simulink model "svpwmmod"  (R2020a)
settings: Solver=ode1  StartTime=0.0  StopTime=0.05  FixedStep=10e-6  MaxStep=0.00001  RelTol=1e-3
InitFcn:
  | Ualf=250;
  | Ubet=250;
  | f=50;
  | fc=5000;
  | Udc=500;
  | T_dead=20e-4
libraries: powerlib x23, dsparch4 x8, simulink x4, powerlib_meascontrol x2
settings Model: Creator=Administrator  LastModifiedBy=DELL
settings SolverCC: AutoInsertRateTranBlk=on
settings DataIOCC: LimitDataPoints=on  SaveFormat=Array  SignalLoggingSaveFormat=ModelDataLogs  ReturnWorkspaceOutputs=off
settings OptimizationCC: ExpressionDepthLimit=2147483647  InitFltsAndDblsToZero=on  LifeSpan=inf
settings DebuggingCC: SaveWithParameterizedLinksMsg=none  UnderspecifiedInitializationDetection=Classic  MergeDetectMultiDrivingBlocksExec=none  SignalResolutionControl=TryResolveAllWithWarning  SolverPrmCheckMsg=warning  MultiTaskDSMMsg=warning  MultiTaskCondExecSysMsg=none  MultiTaskRateTransMsg=warning  FcnCallInpInsideContextMsg=warning  StateNameClashWarn=warning  SFUnexpectedBacktrackingDiag=warning  SFNoUnconditionalDefaultTransitionDiag=warning  ArithmeticOperatorsInVariantConditions=warning
settings HardwareCC: ProdBitPerPointer=32  ProdBitPerSizeT=32  ProdBitPerPtrDiffT=32  ProdLargestAtomicFloat=None  ProdIntDivRoundTo=Undefined  ProdEndianess=Unspecified  ProdWordSize=32  ProdHWDeviceType=32-bit Generic
settings ModelReferenceCC: PropagateSignalLabelsOutOfModel=off
settings SFSimCC: SimUseLocalCustomCode=off  CustomCodeUndefinedFunction=UseInterfaceOnly
settings RTWCC: RTWUseLocalCustomCode=off
settings CodeAppCC: StateflowObjectComments=on
settings GRTTargetCC: TargetFcnLib=ansi_tfl_tmw.mat  TargetLangStandard=C89/C90 (ANSI)  CombineOutputUpdateFcns=off  GRTInterface=on
settings ConfigComp: CovMetricSettings=dw  CovHtmlReporting=on  CovSaveCumulativeToWorkspaceVar=on  CovSaveSingleToWorkspaceVar=on  CovExternalEMLEnable=off

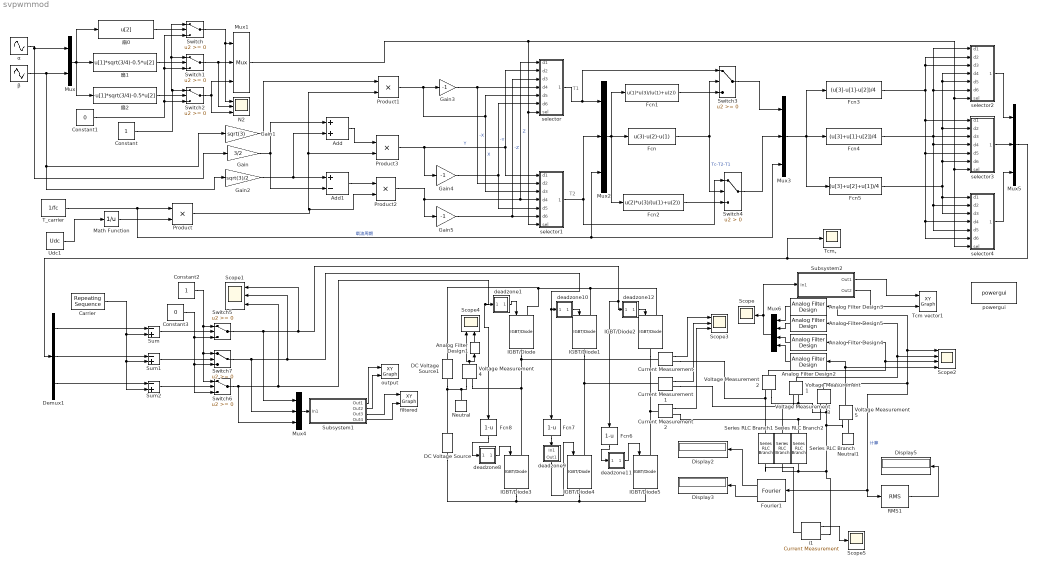
== system svpwmmod ==
  note: T2
  note: T1
  Add : Sum
  Add1 : Sum  Inputs=+-
  Analog Filter Design{1..5} (5 alike) : dsparch4/Analog Filter Design  method=Bessel  filttype=Lowpass  N=4  Wlo=1200  Whi=80  Rp=2  Rs=40
  "Carrier " : simulink/Sources/Repeating Sequence  rep_seq_t=[0 1/(2*fc) 1/(fc)]  rep_seq_y=[0 1/10000 0]
  Constant : Constant
  Constant1 : Constant  Value=0
  Constant2 : Constant
  Constant3 : Constant  Value=0
  Current Measurement : powerlib/Measurements/Current Measurement  PhasorSimulation=off  OutputType=Complex  PSBequivalent=0
  Current Measurement1 : powerlib/Measurements/Current Measurement  PhasorSimulation=off  OutputType=Complex  PSBequivalent=0
  Current Measurement2 : powerlib/Measurements/Current Measurement  PhasorSimulation=off  OutputType=Complex  PSBequivalent=0
  DC Voltage Source : powerlib/Electrical Sources/DC Voltage Source  Amplitude=0.5*(Udc)  Measurements=None
  DC Voltage Source1 : powerlib/Electrical Sources/DC Voltage Source  Amplitude=0.5*(Udc)  Measurements=None
  Demux1 : Demux  Outputs=3
  Display2 : Display
  Display3 : Display
  Display5 : Display
  Fcn : Fcn  Expr=u(3)-u(2)-u(1)
  Fcn1 : Fcn  Expr=u(1)*u(3)/(u(1)+u(2))
  Fcn2 : Fcn  Expr=u(2)*u(3)/(u(1)+u(2))
  Fcn3 : Fcn  Expr=(u[3]-u[1]-u[2])/4
  Fcn4 : Fcn  Expr=(u[3]+u[1]-u[2])/4
  Fcn5 : Fcn  Expr=(u[3]+u[2]+u[1])/4
  Fcn6 : Fcn  Expr=1-u
  Fcn7 : Fcn  Expr=1-u
  Fcn8 : Fcn  Expr=1-u
  Fourier1 : powerlib_meascontrol/Measurements/Fourier  Freq=50  n=1  InInit=[0, 0]  Ts=0
  Gain : Gain  Gain=3/2
  Gain1 : Gain  Gain=sqrt(3)
  Gain2 : Gain  Gain=sqrt(3)/2
  Gain3 : Gain  Gain=-1
  Gain4 : Gain  Gain=-1
  Gain5 : Gain  Gain=-1
  IGBT/Diode{,1..5} (6 alike) : powerlib/Power Electronics/IGBT//Diode  Ron=1e-3  Rs=1e5  Cs=inf  Measurements=off
  Math Function : Math  Operator=reciprocal  SignedPower=on  SaturateOnIntegerOverflow=on
  Mux : Mux  Inputs=2
  Mux{1..5} (5 alike) : Mux  Inputs=3
  Mux6 : Mux
  N2 : Scope  NumInputPorts=3
  Neutral : powerlib/Elements/Neutral  LConnTagsString=a  NodeNumber=10
      settings: SourceProductBaseCode=PS
  Neutral1 : powerlib/Elements/Neutral  LConnTagsString=a  NodeNumber=10
      settings: SourceProductBaseCode=PS
  Product{,1..3} (4 alike) : Product  RndMeth=Zero
  RMS1 : powerlib_meascontrol/Measurements/RMS  TrueRMS=on  Freq=60  RMSInit=120  Ts=0
  Scope : Scope
  Scope1 : Scope  NumInputPorts=3
  Scope2 : Scope  NumInputPorts=4
  Scope3 : Scope  NumInputPorts=3
  Scope4 : Scope  NumInputPorts=2
  Scope5 : Scope
  Series RLC Branch : powerlib/Elements/Series RLC Branch  LConnTagsString=__new0  RConnTagsString=__new0  BranchType=RL  Resistance=10  Inductance=5e-3  SetiL0=off  InitialCurrent=0  Capacitance=1e-6  Setx0=off  InitialVoltage=0  Measurements=None
  Series RLC Branch1 : powerlib/Elements/Series RLC Branch  LConnTagsString=__new0  RConnTagsString=__new0  BranchType=RL  Resistance=10  Inductance=5e-3  SetiL0=off  InitialCurrent=0  Capacitance=1e-6  Setx0=off  InitialVoltage=0  Measurements=None
  Series RLC Branch2 : powerlib/Elements/Series RLC Branch  LConnTagsString=__new0  RConnTagsString=__new0  BranchType=RL  Resistance=10  Inductance=5e-3  SetiL0=off  InitialCurrent=0  Capacitance=1e-6  Setx0=off  InitialVoltage=0  Measurements=None
  Subsystem1 : Subsystem
  Subsystem2 : Subsystem
  Sum : Sum  Inputs=-+  SaturateOnIntegerOverflow=on
  Sum1 : Sum  Inputs=-+  SaturateOnIntegerOverflow=on
  Sum2 : Sum  Inputs=-+  SaturateOnIntegerOverflow=on
  Switch{,1..3} (4 alike) : Switch
  Switch4 : Switch  Criteria=u2 > Threshold
  Switch5 : Switch  SaturateOnIntegerOverflow=on
  Switch6 : Switch  SaturateOnIntegerOverflow=on
  Switch7 : Switch  SaturateOnIntegerOverflow=on
  T_carrier : Constant  Value=1/fc
  Tcm vector1 : simulink/Sinks/XY Graph  xmin=-400  xmax=400  ymin=-400  ymax=400  st=-1
  Tcm。 : Scope
  Udc1 : Constant  Value=Udc
  Voltage Measurement{1..5} (5 alike) : powerlib/Measurements/Voltage Measurement  PhasorSimulation=off  OutputType=Complex  PSBequivalent=0
  deadzone1 : Subsystem
  deadzone10 : Subsystem
  deadzone11 : Subsystem
  deadzone12 : Subsystem
  deadzone8 : Subsystem
  deadzone9 : Subsystem
  filtered : simulink/Sinks/XY Graph  xmin=-1  xmax=1  ymin=-1  ymax=1  st=-1
  i1 : powerlib/Measurements/Current Measurement  PhasorSimulation=off  OutputType=Complex  PSBequivalent=0
  output : simulink/Sinks/XY Graph  xmin=-1  xmax=1  ymin=-1  ymax=1  st=-1
  powergui : powerlib/powergui  Priority=1  SimulationMode=Discrete  SampleTime=50e-6  frequency=60  Iterations=50  frequencyindice=0  Pbase=100e6  ErrMax=1e-4  UnitsV=kV  UnitsW=MW  buscounter=0  FunctionMessages=off  echomessages=off  EnableUseOfTLC=off  CurrentSourceSwitches=off  DisableSnubberDevices=off  DisableRonSwitches=off  DisableVfSwitches=off  DisplayEquations=off  AutomaticDiscreteSolvers=off  SolverType=Tustin/Backward Euler (TBE)  Interpol=off  ExternalGateDelay=off  methode=off  Ts=100  x0status=blocks  SPID=off  SwTol=0  HookPort=off  NonlinearTolerance=1e-4  nMaxIteration=100  ContinueOnMaxIteration=off  RestoreLinks=warning  ResistiveCurrentMeasurement=off  Frange=[0:2:500]  Ylog=off  Xlog=on  ShowGrid=off  save=off  variable=ZData  structure=output  ZoomFFT=off  StartTime=0.02  cycles=1  DisplayStyle=1  fundamental=60  FreqAxis=off  MaxFrequency=1000  frequencyindicesteady=1  RmsSteady=1  display=off
  selector : Subsystem
  selector1 : Subsystem
  selector2 : Subsystem
  selector3 : Subsystem
  selector4 : Subsystem
  α : Sin  Amplitude=Ualf  Frequency=f*2*pi  Phase=pi/2  SampleTime=0
  β : Sin  Amplitude=Ubet  Frequency=f*2*pi  SampleTime=0
  扇0 : Fcn  Expr=u[2]
  扇1 : Fcn  Expr=u[1]*sqrt(3/4)-0.5*u[2]
  扇2 : Fcn  Expr=-u[1]*sqrt(3/4)-0.5*u[2]
  wires:
  Constant/1 -> Switch2/1, Switch/1, Switch1/1
  扇1/1 -> Switch1/2
  Switch2/1 -> Mux1/3, N2/3
  扇0/1 -> Switch/2
  Constant1/1 -> Switch/3, Switch1/3, Switch2/3
  Mux/1 -> 扇2/1, 扇1/1, 扇0/1
  Switch/1 -> N2/1, Mux1/1
  Switch1/1 -> Mux1/2, N2/2
  Mux1/1 -> selector4/7(sel), selector3/7(sel), selector2/7(sel), selector/7(sel), selector1/7(sel)
  扇2/1 -> Switch2/2
  Udc1/1 -> Math Function/1
  Add/1 -> Product3/1
  Add1/1 -> Product2/1
  Gain1/1 -> Product1/1
  Gain/1 -> Add/1, Add1/2
  Math Function/1 -> Product/2
  Product/1 -> Product1/2, Product3/2, Product2/2
  Gain2/1 -> Add/2, Add1/1
  selector1/1(Out1) -> Mux2/2, Switch4/1
  Gain4/1 -> selector1/5(d5), selector/6(d6)  "-Y"
  Product2/1 -> Gain5/1, selector/1(d1), selector1/4(d4)  "Z"
  Product1/1 -> selector1/3(d3), selector/5(d5), Gain3/1  "X"
  Fcn2/1 -> Switch4/3
  Gain3/1 -> selector1/2(d2), selector/4(d4)  "-X"
  Gain5/1 -> selector1/6(d6), selector/3(d3)  "-Z"
  Fcn1/1 -> Switch3/3
  Fcn/1 -> Switch4/2, Switch3/2  "Tc-T2-T1"
  Product3/1 -> Gain4/1, selector1/1(d1), selector/2(d2)  "Y"
  selector3/1(Out1) -> Mux5/2
  selector2/1(Out1) -> Mux5/1
  selector4/1(Out1) -> Mux5/3
  Fcn5/1 -> selector3/2(d2), selector2/4(d4), selector2/5(d5), selector3/6(d6), selector4/1(d1), selector4/3(d3)
  Demux1/3 -> Sum2/1
  Demux1/1 -> Sum/1
  Demux1/2 -> Sum1/1
  Sum1/1 -> Switch7/2
  Sum/1 -> Switch5/2
  Constant2/1 -> Switch5/1, Switch7/1, Switch6/1
  Sum2/1 -> Switch6/2
  Constant3/1 -> Switch6/3, Switch7/3, Switch5/3
  Mux5/1 -> Tcm。/1, Demux1/1
  "Carrier "/1 -> Sum/2, Sum1/2, Sum2/2
  Mux2/1 -> Fcn2/1, Fcn1/1, Fcn/1
  T_carrier/1 -> Mux2/3, Mux3/3, Product/1  "载波周期"
  Switch3/1 -> Mux3/1
  Switch4/1 -> Mux3/2
  Mux3/1 -> Fcn5/1, Fcn4/1, Fcn3/1
  Subsystem1/1(Out1) -> output/1
  Subsystem1/2(Out2) -> output/2
  Mux4/1 -> Subsystem1/1(In1)
  Subsystem1/3(Out3) -> filtered/1
  Subsystem1/4(Out4) -> filtered/2
  RMS1/1 -> Display5/1
  Voltage Measurement3/1 -> RMS1/1, Fourier1/1, Scope2/1, Analog Filter Design3/1  "计算"
  Fourier1/1 -> Display2/1
  Fourier1/2 -> Display3/1
  Mux6/1 -> Subsystem2/1(In1), Scope/1
  Subsystem2/1(Out1) -> Tcm vector1/1
  Subsystem2/2(Out2) -> Tcm vector1/2
  Analog Filter Design3/1 -> Mux6/1
  Analog Filter Design4/1 -> Mux6/3
  Analog Filter Design5/1 -> Mux6/2
  Voltage Measurement2/1 -> Scope2/3, Analog Filter Design4/1
  Voltage Measurement1/1 -> Scope2/2, Analog Filter Design5/1
  Switch7/1 -> Scope1/2, deadzone10/1(In1), Fcn7/1, Mux4/2
  Switch5/1 -> Scope1/1, deadzone12/1(In1), Fcn6/1, Mux4/1
  α/1 -> Mux/1, Gain/1
  β/1 -> Gain2/1, Gain1/1, Mux/2
  Current Measurement/1 -> Scope3/1
  Current Measurement1/1 -> Scope3/2
  Current Measurement2/1 -> Scope3/3
  selector/1(Out1) -> Switch3/1, Mux2/1
  Fcn3/1 -> selector3/1(d1), selector4/4(d4), selector4/6(d6), selector3/5(d5), selector2/2(d2), selector2/3(d3)
  Fcn4/1 -> selector4/2(d2), selector4/5(d5), selector3/4(d4), selector3/3(d3), selector2/1(d1), selector2/6(d6)
  Voltage Measurement4/1 -> Analog Filter Design1/1, Scope4/1
  Analog Filter Design1/1 -> Scope4/2
  Analog Filter Design2/1 -> Mux6/4
  Voltage Measurement5/1 -> Scope2/4, Analog Filter Design2/1
  deadzone1/1(Out1) -> IGBT/Diode/1
  Switch6/1 -> deadzone1/1(In1), Fcn8/1, Scope1/3, Mux4/3
  Fcn8/1 -> deadzone8/1(In1)
  Fcn7/1 -> deadzone9/1(In1)
  deadzone9/1(Out1) -> IGBT/Diode4/1
  deadzone10/1(Out1) -> IGBT/Diode1/1
  Fcn6/1 -> deadzone11/1(In1)
  deadzone11/1(Out1) -> IGBT/Diode5/1
  deadzone12/1(Out1) -> IGBT/Diode2/1
  deadzone8/1(Out1) -> IGBT/Diode3/1
  i1/1 -> Scope5/1
  connections:
  IGBT/Diode/LConn1 -- DC Voltage Source1/RConn1 -- IGBT/Diode2/LConn1 -- IGBT/Diode1/LConn1
  Voltage Measurement2/LConn1 -- Current Measurement/RConn1 -- Series RLC Branch1/LConn1
  IGBT/Diode2/RConn1 -- Current Measurement2/LConn1 -- IGBT/Diode5/LConn1
  IGBT/Diode3/RConn1 -- DC Voltage Source/LConn1 -- IGBT/Diode5/RConn1 -- IGBT/Diode4/RConn1
  IGBT/Diode1/RConn1 -- Current Measurement1/LConn1 -- IGBT/Diode4/LConn1
  DC Voltage Source1/LConn1 -- Neutral/LConn1 -- Voltage Measurement4/LConn2 -- DC Voltage Source/RConn1
  Series RLC Branch2/RConn1 -- Voltage Measurement5/LConn1 -- Voltage Measurement2/LConn2 -- Voltage Measurement1/LConn2 -- Voltage Measurement3/LConn2 -- i1/RConn1 -- Series RLC Branch/RConn1
  IGBT/Diode/RConn1 -- Current Measurement/LConn1 -- Voltage Measurement4/LConn1 -- IGBT/Diode3/LConn1
  Voltage Measurement1/LConn1 -- Current Measurement1/RConn1 -- Series RLC Branch2/LConn1
  Voltage Measurement3/LConn1 -- Current Measurement2/RConn1 -- Series RLC Branch/LConn1
  Neutral1/LConn1 -- Voltage Measurement5/LConn2
  Series RLC Branch1/RConn1 -- i1/LConn1

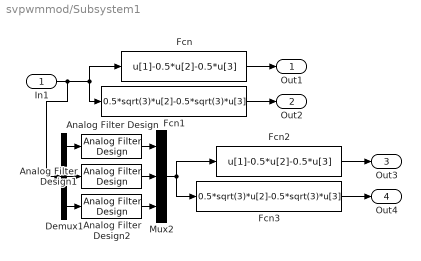
== system svpwmmod/Subsystem1 ==
  In1 : Inport
  Analog Filter Design : dsparch4/Analog Filter Design  method=Bessel  filttype=Lowpass  N=3  Wlo=1200  Whi=80  Rp=2  Rs=40
  Analog Filter Design1 : dsparch4/Analog Filter Design  method=Bessel  filttype=Lowpass  N=3  Wlo=1200  Whi=80  Rp=2  Rs=40
  Analog Filter Design2 : dsparch4/Analog Filter Design  method=Bessel  filttype=Lowpass  N=3  Wlo=1200  Whi=80  Rp=2  Rs=40
  Demux1 : Demux  Outputs=3
  Fcn : Fcn  Expr=u[1]-0.5*u[2]-0.5*u[3]
  Fcn1 : Fcn  Expr=0.5*sqrt(3)*u[2]-0.5*sqrt(3)*u[3]
  Fcn2 : Fcn  Expr=u[1]-0.5*u[2]-0.5*u[3]
  Fcn3 : Fcn  Expr=0.5*sqrt(3)*u[2]-0.5*sqrt(3)*u[3]
  Mux2 : Mux  Inputs=3
  Out1 : Outport  VectorParamsAs1DForOutWhenUnconnected=off
  Out2 : Outport  Port=2  VectorParamsAs1DForOutWhenUnconnected=off
  Out3 : Outport  Port=3  VectorParamsAs1DForOutWhenUnconnected=off
  Out4 : Outport  Port=4  VectorParamsAs1DForOutWhenUnconnected=off
  wires:
  Fcn/1 -> Out1/1
  Fcn1/1 -> Out2/1
  In1/1 -> Demux1/1, Fcn/1, Fcn1/1
  Fcn3/1 -> Out4/1
  Fcn2/1 -> Out3/1
  Demux1/1 -> Analog Filter Design/1
  Demux1/2 -> Analog Filter Design1/1
  Demux1/3 -> Analog Filter Design2/1
  Analog Filter Design/1 -> Mux2/1
  Analog Filter Design1/1 -> Mux2/2
  Analog Filter Design2/1 -> Mux2/3
  Mux2/1 -> Fcn3/1, Fcn2/1

== system svpwmmod/Subsystem2 ==
  In1 : Inport
  Fcn : Fcn  Expr=u[1]-0.5*u[2]-0.5*u[3]
  Fcn1 : Fcn  Expr=0.5*sqrt(3)*u[2]-0.5*sqrt(3)*u[3]
  Out1 : Outport  VectorParamsAs1DForOutWhenUnconnected=off
  Out2 : Outport  Port=2  VectorParamsAs1DForOutWhenUnconnected=off
  wires:
  Fcn/1 -> Out1/1
  Fcn1/1 -> Out2/1
  In1/1 -> Fcn/1, Fcn1/1

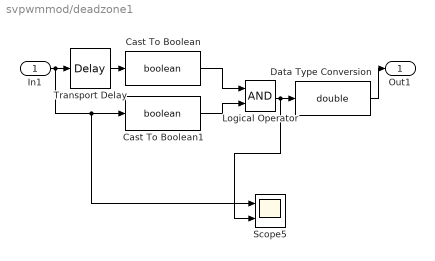
== system svpwmmod/deadzone1 ==
  In1 : Inport
  Cast To Boolean : DataTypeConversion  OutDataTypeStr=boolean
  Cast To Boolean1 : DataTypeConversion  OutDataTypeStr=boolean
  Data Type Conversion : DataTypeConversion  OutDataTypeStr=double
  Logical Operator : Logic  AllPortsSameDT=off  OutDataTypeStr=boolean
  Scope5 : Scope  NumInputPorts=2
  Transport Delay : TransportDelay  DelayTime=T_dead
  Out1 : Outport  VectorParamsAs1DForOutWhenUnconnected=off
  wires:
  Transport Delay/1 -> Cast To Boolean/1
  Cast To Boolean/1 -> Logical Operator/1
  Cast To Boolean1/1 -> Logical Operator/2
  In1/1 -> Scope5/1, Cast To Boolean1/1, Transport Delay/1
  Data Type Conversion/1 -> Out1/1
  Logical Operator/1 -> Scope5/2, Data Type Conversion/1

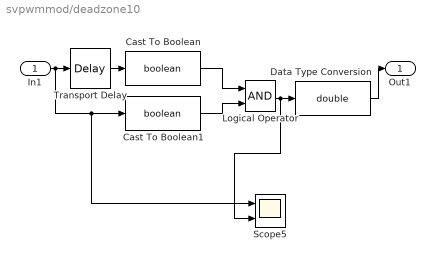
== system svpwmmod/deadzone10 ==
  In1 : Inport
  Cast To Boolean : DataTypeConversion  OutDataTypeStr=boolean
  Cast To Boolean1 : DataTypeConversion  OutDataTypeStr=boolean
  Data Type Conversion : DataTypeConversion  OutDataTypeStr=double
  Logical Operator : Logic  AllPortsSameDT=off  OutDataTypeStr=boolean
  Scope5 : Scope  NumInputPorts=2
  Transport Delay : TransportDelay  DelayTime=T_dead
  Out1 : Outport  VectorParamsAs1DForOutWhenUnconnected=off
  wires:
  Transport Delay/1 -> Cast To Boolean/1
  Cast To Boolean/1 -> Logical Operator/1
  Cast To Boolean1/1 -> Logical Operator/2
  In1/1 -> Scope5/1, Cast To Boolean1/1, Transport Delay/1
  Data Type Conversion/1 -> Out1/1
  Logical Operator/1 -> Scope5/2, Data Type Conversion/1

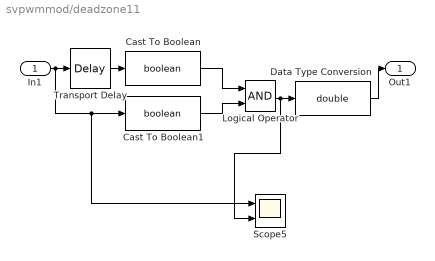
== system svpwmmod/deadzone11 ==
  In1 : Inport
  Cast To Boolean : DataTypeConversion  OutDataTypeStr=boolean
  Cast To Boolean1 : DataTypeConversion  OutDataTypeStr=boolean
  Data Type Conversion : DataTypeConversion  OutDataTypeStr=double
  Logical Operator : Logic  AllPortsSameDT=off  OutDataTypeStr=boolean
  Scope5 : Scope  NumInputPorts=2
  Transport Delay : TransportDelay  DelayTime=T_dead
  Out1 : Outport  VectorParamsAs1DForOutWhenUnconnected=off
  wires:
  Transport Delay/1 -> Cast To Boolean/1
  Cast To Boolean/1 -> Logical Operator/1
  Cast To Boolean1/1 -> Logical Operator/2
  In1/1 -> Scope5/1, Cast To Boolean1/1, Transport Delay/1
  Data Type Conversion/1 -> Out1/1
  Logical Operator/1 -> Scope5/2, Data Type Conversion/1

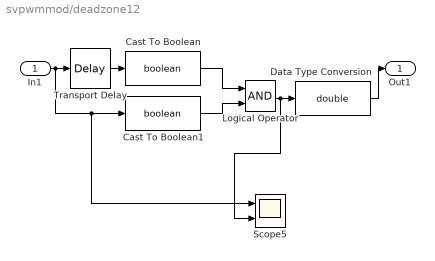
== system svpwmmod/deadzone12 ==
  In1 : Inport
  Cast To Boolean : DataTypeConversion  OutDataTypeStr=boolean
  Cast To Boolean1 : DataTypeConversion  OutDataTypeStr=boolean
  Data Type Conversion : DataTypeConversion  OutDataTypeStr=double
  Logical Operator : Logic  AllPortsSameDT=off  OutDataTypeStr=boolean
  Scope5 : Scope  NumInputPorts=2
  Transport Delay : TransportDelay  DelayTime=T_dead
  Out1 : Outport  VectorParamsAs1DForOutWhenUnconnected=off
  wires:
  Transport Delay/1 -> Cast To Boolean/1
  Cast To Boolean/1 -> Logical Operator/1
  Cast To Boolean1/1 -> Logical Operator/2
  In1/1 -> Scope5/1, Cast To Boolean1/1, Transport Delay/1
  Data Type Conversion/1 -> Out1/1
  Logical Operator/1 -> Scope5/2, Data Type Conversion/1

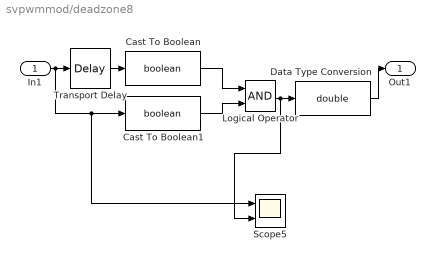
== system svpwmmod/deadzone8 ==
  In1 : Inport
  Cast To Boolean : DataTypeConversion  OutDataTypeStr=boolean
  Cast To Boolean1 : DataTypeConversion  OutDataTypeStr=boolean
  Data Type Conversion : DataTypeConversion  OutDataTypeStr=double
  Logical Operator : Logic  AllPortsSameDT=off  OutDataTypeStr=boolean
  Scope5 : Scope  NumInputPorts=2
  Transport Delay : TransportDelay  DelayTime=T_dead
  Out1 : Outport  VectorParamsAs1DForOutWhenUnconnected=off
  wires:
  Transport Delay/1 -> Cast To Boolean/1
  Cast To Boolean/1 -> Logical Operator/1
  Cast To Boolean1/1 -> Logical Operator/2
  In1/1 -> Scope5/1, Cast To Boolean1/1, Transport Delay/1
  Data Type Conversion/1 -> Out1/1
  Logical Operator/1 -> Scope5/2, Data Type Conversion/1

== system svpwmmod/deadzone9 ==
  In1 : Inport
  Cast To Boolean : DataTypeConversion  OutDataTypeStr=boolean
  Cast To Boolean1 : DataTypeConversion  OutDataTypeStr=boolean
  Data Type Conversion : DataTypeConversion  OutDataTypeStr=double
  Logical Operator : Logic  AllPortsSameDT=off  OutDataTypeStr=boolean
  Scope5 : Scope  NumInputPorts=2
  Transport Delay : TransportDelay  DelayTime=T_dead
  Out1 : Outport  VectorParamsAs1DForOutWhenUnconnected=off
  wires:
  Transport Delay/1 -> Cast To Boolean/1
  Cast To Boolean/1 -> Logical Operator/1
  Cast To Boolean1/1 -> Logical Operator/2
  In1/1 -> Scope5/1, Cast To Boolean1/1, Transport Delay/1
  Data Type Conversion/1 -> Out1/1
  Logical Operator/1 -> Scope5/2, Data Type Conversion/1

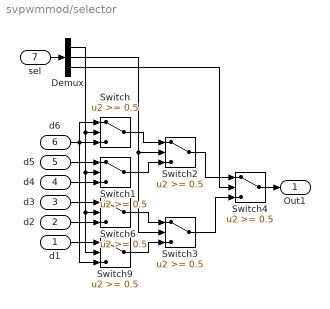
== system svpwmmod/selector ==
  d1 : Inport
  d2 : Inport  Port=2
  d3 : Inport  Port=3
  d4 : Inport  Port=4
  d5 : Inport  Port=5
  d6 : Inport  Port=6
  sel : Inport  Port=7
  Demux : Demux  Outputs=3
  Switch{,1..4,6,9} (7 alike) : Switch  Threshold=0.5
  Out1 : Outport  VectorParamsAs1DForOutWhenUnconnected=off
  wires:
  d6/1 -> Switch9/3, Switch/1, Switch/3
  d5/1 -> Switch1/1
  d4/1 -> Switch1/3
  d2/1 -> Switch6/3
  d3/1 -> Switch6/1
  Switch/1 -> Switch2/1
  Switch1/1 -> Switch2/3
  Switch6/1 -> Switch3/1
  Switch9/1 -> Switch3/3
  Switch2/1 -> Switch4/1
  Switch3/1 -> Switch4/3
  Switch4/1 -> Out1/1
  sel/1 -> Demux/1
  Demux/1 -> Switch/2, Switch1/2, Switch6/2, Switch9/2
  Demux/2 -> Switch2/2, Switch3/2
  Demux/3 -> Switch4/2
  d1/1 -> Switch9/1

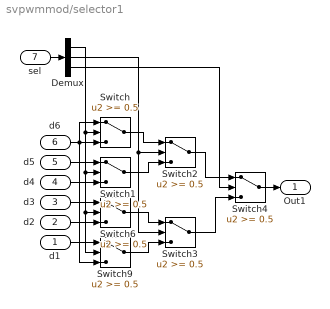
== system svpwmmod/selector1 ==
  d1 : Inport
  d2 : Inport  Port=2
  d3 : Inport  Port=3
  d4 : Inport  Port=4
  d5 : Inport  Port=5
  d6 : Inport  Port=6
  sel : Inport  Port=7
  Demux : Demux  Outputs=3
  Switch{,1..4,6,9} (7 alike) : Switch  Threshold=0.5
  Out1 : Outport  VectorParamsAs1DForOutWhenUnconnected=off
  wires:
  d6/1 -> Switch9/3, Switch/1, Switch/3
  d5/1 -> Switch1/1
  d4/1 -> Switch1/3
  d2/1 -> Switch6/3
  d3/1 -> Switch6/1
  Switch/1 -> Switch2/1
  Switch1/1 -> Switch2/3
  Switch6/1 -> Switch3/1
  Switch9/1 -> Switch3/3
  Switch2/1 -> Switch4/1
  Switch3/1 -> Switch4/3
  Switch4/1 -> Out1/1
  sel/1 -> Demux/1
  Demux/1 -> Switch/2, Switch1/2, Switch6/2, Switch9/2
  Demux/2 -> Switch2/2, Switch3/2
  Demux/3 -> Switch4/2
  d1/1 -> Switch9/1

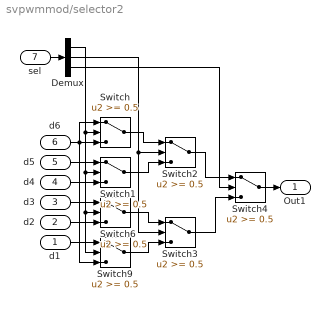
== system svpwmmod/selector2 ==
  d1 : Inport
  d2 : Inport  Port=2
  d3 : Inport  Port=3
  d4 : Inport  Port=4
  d5 : Inport  Port=5
  d6 : Inport  Port=6
  sel : Inport  Port=7
  Demux : Demux  Outputs=3
  Switch{,1..4,6,9} (7 alike) : Switch  Threshold=0.5
  Out1 : Outport  VectorParamsAs1DForOutWhenUnconnected=off
  wires:
  d6/1 -> Switch9/3, Switch/1, Switch/3
  d5/1 -> Switch1/1
  d4/1 -> Switch1/3
  d2/1 -> Switch6/3
  d3/1 -> Switch6/1
  Switch/1 -> Switch2/1
  Switch1/1 -> Switch2/3
  Switch6/1 -> Switch3/1
  Switch9/1 -> Switch3/3
  Switch2/1 -> Switch4/1
  Switch3/1 -> Switch4/3
  Switch4/1 -> Out1/1
  sel/1 -> Demux/1
  Demux/1 -> Switch/2, Switch1/2, Switch6/2, Switch9/2
  Demux/2 -> Switch2/2, Switch3/2
  Demux/3 -> Switch4/2
  d1/1 -> Switch9/1

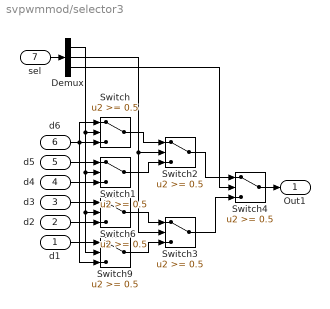
== system svpwmmod/selector3 ==
  d1 : Inport
  d2 : Inport  Port=2
  d3 : Inport  Port=3
  d4 : Inport  Port=4
  d5 : Inport  Port=5
  d6 : Inport  Port=6
  sel : Inport  Port=7
  Demux : Demux  Outputs=3
  Switch{,1..4,6,9} (7 alike) : Switch  Threshold=0.5
  Out1 : Outport  VectorParamsAs1DForOutWhenUnconnected=off
  wires:
  d6/1 -> Switch9/3, Switch/1, Switch/3
  d5/1 -> Switch1/1
  d4/1 -> Switch1/3
  d2/1 -> Switch6/3
  d3/1 -> Switch6/1
  Switch/1 -> Switch2/1
  Switch1/1 -> Switch2/3
  Switch6/1 -> Switch3/1
  Switch9/1 -> Switch3/3
  Switch2/1 -> Switch4/1
  Switch3/1 -> Switch4/3
  Switch4/1 -> Out1/1
  sel/1 -> Demux/1
  Demux/1 -> Switch/2, Switch1/2, Switch6/2, Switch9/2
  Demux/2 -> Switch2/2, Switch3/2
  Demux/3 -> Switch4/2
  d1/1 -> Switch9/1

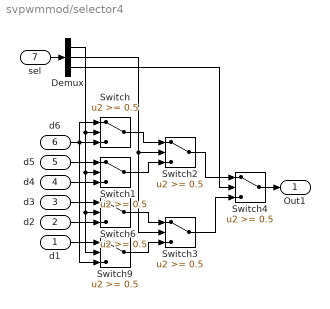
== system svpwmmod/selector4 ==
  d1 : Inport
  d2 : Inport  Port=2
  d3 : Inport  Port=3
  d4 : Inport  Port=4
  d5 : Inport  Port=5
  d6 : Inport  Port=6
  sel : Inport  Port=7
  Demux : Demux  Outputs=3
  Switch{,1..4,6,9} (7 alike) : Switch  Threshold=0.5
  Out1 : Outport  VectorParamsAs1DForOutWhenUnconnected=off
  wires:
  d6/1 -> Switch9/3, Switch/1, Switch/3
  d5/1 -> Switch1/1
  d4/1 -> Switch1/3
  d2/1 -> Switch6/3
  d3/1 -> Switch6/1
  Switch/1 -> Switch2/1
  Switch1/1 -> Switch2/3
  Switch6/1 -> Switch3/1
  Switch9/1 -> Switch3/3
  Switch2/1 -> Switch4/1
  Switch3/1 -> Switch4/3
  Switch4/1 -> Out1/1
  sel/1 -> Demux/1
  Demux/1 -> Switch/2, Switch1/2, Switch6/2, Switch9/2
  Demux/2 -> Switch2/2, Switch3/2
  Demux/3 -> Switch4/2
  d1/1 -> Switch9/1
